simulink model "ZN_FrequencyTuning"  (Simulink 10.3)
settings: Solver=VariableStepAuto  StartTime=0.0  StopTime=10.0  MaxStep=0.01  RelTol=1e-3
settings Model: Creator=Mertcan  LastModifiedBy=Mertcan
settings SolverCC: AlgebraicLoopSolver=Auto
settings DataIOCC: SaveFormat=Dataset  SignalLoggingSaveFormat=Dataset  ReturnWorkspaceOutputs=on
settings OptimizationCC: ExpressionDepthLimit=128  LifeSpan=auto
settings DebuggingCC: UnderspecifiedInitializationDetection=Simplified  MergeDetectMultiDrivingBlocksExec=error  FcnCallInpInsideContextMsg=error  StateNameClashWarn=none  SFUnexpectedBacktrackingDiag=error  SFNoUnconditionalDefaultTransitionDiag=error  SFExecutionAtInitializationDiag=warning  SFMachineParentedDataDiag=error  ArithmeticOperatorsInVariantConditions=error
settings HardwareCC: ProdBitPerPointer=64  ProdBitPerSizeT=64  ProdBitPerPtrDiffT=64  ProdLargestAtomicFloat=Float  ProdIntDivRoundTo=Zero  ProdEndianess=LittleEndian  ProdWordSize=64  ProdHWDeviceType=Intel->x86-64 (Windows64)
settings ModelReferenceCC: PropagateSignalLabelsOutOfModel=on
settings SFSimCC: SimUseLocalCustomCode=on  CustomCodeUndefinedFunction=FilterOut
settings RTWCC: RTWUseLocalCustomCode=on
settings CodeAppCC: StateflowObjectComments=off
settings GRTTargetCC: TargetLangStandard=C99 (ISO)  CombineOutputUpdateFcns=on  GRTInterface=off
settings ConfigComp: CovMetricSettings=dwe  CovSaveCumulativeToWorkspaceVar=off  CovSaveSingleToWorkspaceVar=off  CovExternalEMLEnable=on

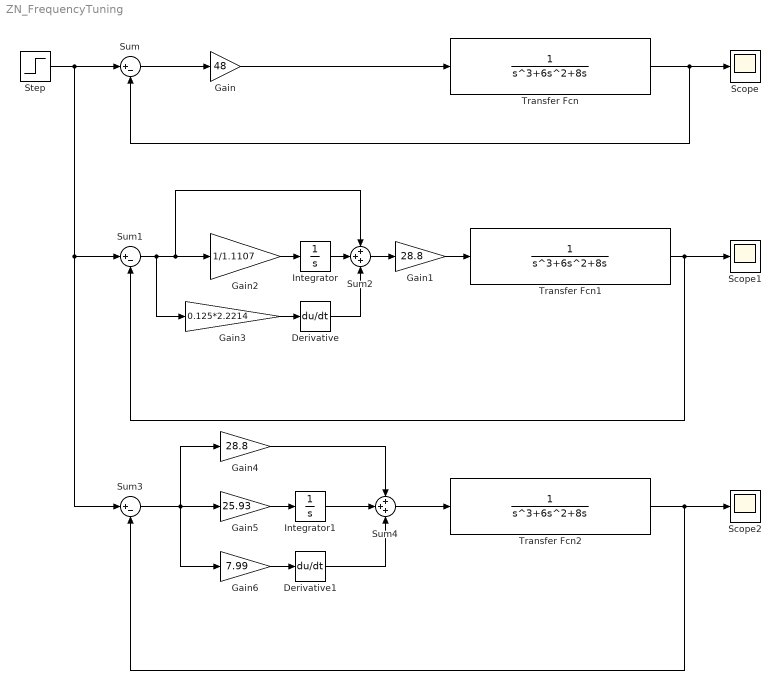
== system ZN_FrequencyTuning ==
  Derivative : Derivative
  Derivative1 : Derivative
  Gain : Gain  Gain=48
  Gain1 : Gain  Gain=28.8
  Gain2 : Gain  Gain=1/1.1107
  Gain3 : Gain  Gain=0.125*2.2214
  Gain4 : Gain  Gain=28.8
  Gain5 : Gain  Gain=25.93
  Gain6 : Gain  Gain=7.99
  Integrator : Integrator
  Integrator1 : Integrator
  Scope : Scope
  Scope1 : Scope
  Scope2 : Scope
  Step : Step  Time=0  SampleTime=0
  Sum : Sum  Inputs=|+-
  Sum1 : Sum  Inputs=|+-
  Sum2 : Sum  Inputs=+++
  Sum3 : Sum  Inputs=|+-
  Sum4 : Sum  Inputs=+++
  Transfer Fcn : TransferFcn  Denominator=[1 6 8 0]
  Transfer Fcn1 : TransferFcn  Denominator=[1 6 8 0]
  Transfer Fcn2 : TransferFcn  Denominator=[1 6 8 0]
  wires:
  Sum/1 -> Gain/1
  Gain/1 -> Transfer Fcn/1
  Transfer Fcn/1 -> Scope/1, Sum/2
  Transfer Fcn1/1 -> Sum1/2, Scope1/1
  Gain2/1 -> Integrator/1
  Integrator/1 -> Sum2/2
  Gain3/1 -> Derivative/1
  Derivative/1 -> Sum2/3
  Sum3/1 -> Gain6/1, Gain5/1, Gain4/1
  Derivative1/1 -> Sum4/3
  Gain6/1 -> Derivative1/1
  Integrator1/1 -> Sum4/2
  Gain5/1 -> Integrator1/1
  Gain4/1 -> Sum4/1
  Sum4/1 -> Transfer Fcn2/1
  Transfer Fcn2/1 -> Scope2/1, Sum3/2
  Sum2/1 -> Gain1/1
  Gain1/1 -> Transfer Fcn1/1
  Sum1/1 -> Sum2/1, Gain2/1, Gain3/1
  Step/1 -> Sum3/1, Sum1/1, Sum/1
